simulink model "kalman_verify_v1"  (R2023b)
settings: Solver=VariableStepAuto  StartTime=0.0  StopTime=30  RelTol=1e-3
undefined symbols (not defined in the file): DiscIntNeverNeededParam
libraries: dspsrcs4 x2, simulink x1
settings Model: Creator=Zian Liu  LastModifiedBy=Zian Liu

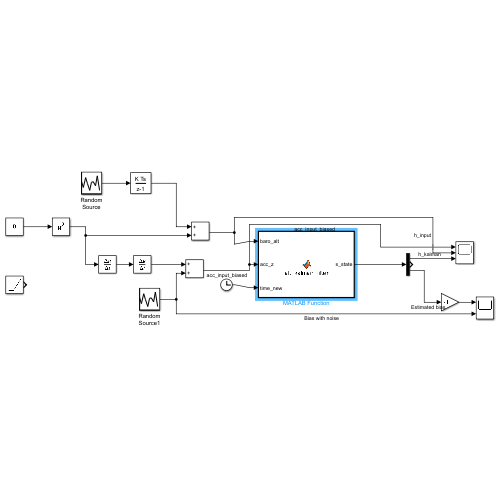
[thumbnail: Simulink's stored preview of the top-level diagram]
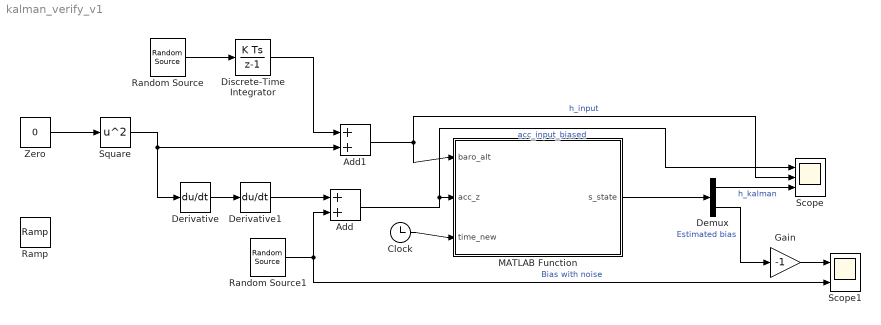
== system kalman_verify_v1 ==
  Add : Sum
  Add1 : Sum
  Clock : Clock
  Demux : Demux  Outputs=3
  Derivative : Derivative
  Derivative1 : Derivative
  Discrete-Time Integrator : DiscreteIntegrator  SampleTime=-1  ICPrevOutput=DiscIntNeverNeededParam  ICPrevScaledInput=DiscIntNeverNeededParam
  Gain : Gain  Gain=-1
  MATLAB Function : MATLAB Function  TreatAsAtomicUnit=on
  Ramp : simulink/Sources/Ramp  slope=0.1  start=0  InitialOutput=0
  Random Source : dspsrcs4/Random Source  SrcType=Gaussian  NormMethod=Ziggurat  CltLength=12  MinVal=0  MaxVal=1  MeanVal=0  VarVal=0.05  RepMode=Not repeatable  rawSeed=1  IsInherit=off  SampMode=Discrete  SampTime=1e-3  SampFrame=1  DataType=Double  OutComplex=Real  OutputFrames=off
  Random Source1 : dspsrcs4/Random Source  SrcType=Gaussian  NormMethod=Ziggurat  CltLength=12  MinVal=0  MaxVal=1  MeanVal=-0.5  VarVal=0.02  RepMode=Not repeatable  rawSeed=1  IsInherit=off  SampMode=Discrete  SampTime=1e-2  SampFrame=1  DataType=Double  OutComplex=Real  OutputFrames=off
  Scope : Scope  NumInputPorts=3
  Scope1 : Scope  NumInputPorts=2
  Square : Math  Operator=square
  Zero : Constant  Value=0  OutDataTypeStr=Inherit: Inherit via back propagation
  wires:
  MATLAB Function/1(s_state) -> Demux/1
  Clock/1 -> MATLAB Function/3(time_new)
  Square/1 -> Derivative/1, Add1/2
  Derivative/1 -> Derivative1/1
  Demux/1 -> Scope/3  "h_kalman"
  Random Source1/1 -> Add/2, Scope1/2  "Bias with noise"
  Add1/1 -> Scope/2, MATLAB Function/1(baro_alt)  "h_input"
  Random Source/1 -> Discrete-Time Integrator/1
  Demux/3 -> Gain/1  "Estimated bias"
  Gain/1 -> Scope1/1
  Add/1 -> Scope/1, MATLAB Function/2(acc_z)  "acc_input_biased"
  Derivative1/1 -> Add/1
  Zero/1 -> Square/1
  Discrete-Time Integrator/1 -> Add1/1

== matlab function kalman_verify_v1/MATLAB Function ==
  data: baro_alt input; s_state output; acc_z input; time_new input
function s_state = alt_kalman_filter(baro_alt, acc_z, time_new)
    % States: {altitude, vertical speed, -bias}
    % Estimated bias is negative such that the first state can converge to the sensor value

    % Declare persistent variables
    persistent s_state_prev P_prev time_old;
    
    % Initialize persistent variables if they are empty
    if isempty(s_state_prev)
        s_state_prev = zeros(3, 1);  % [position; velocity]
        P_prev = diag([0.01 0.01 0.1]);       % Initial covariance matrix with some uncertainty
        time_old = 0;                % Initialize previous time
    end

    % Time step
    dt = time_new - time_old;
    time_old = time_new;
    
    % Kalman filter step
    % State transition matrix
    F = [1, dt, 0.5 * dt^2;
         0, 1, dt;
         0, 0, 1];
    
    % Control input matrix
    G = [0.5 * dt^2;
         dt;
         0];
    
    % Measurement matrix
    H = [1, 0, 0];
    
    % Process noise covariance matrix
    acc_std = 0.1;       % Acceleration noise standard deviation
    Q = G * G' * acc_std^2;
    
    % Measurement noise covariance
    R = 1;             % Measurement noise covariance
    
    % Prediction step
    s_state_pred = F * s_state_prev + G * acc_z;
    P_pred = F * P_prev * F' + Q;
    
    % Update step
    L = H * P_pred * H' + R;
    K = P_pred * H' / L;
    
    % Innovation
    innov = baro_alt - H * s_state_pred;
    
    % State update
    s_state = s_state_pred + K * innov;
    
    % Covariance update
    P = (eye(3) - K * H) * P_pred;
    
    % Update persistent variables for the next iteration
    s_state_prev = s_state;
    P_prev = P;
end
